simulink model "TransformadaZ"  (R2017b)
settings: Solver=ode4  StartTime=0.0  StopTime=10.0  FixedStep=0.0001  RelTol=1e-3
settings Model: Creator=Benjamin Nicolas  LastModifiedBy=Benjamin Nicolas

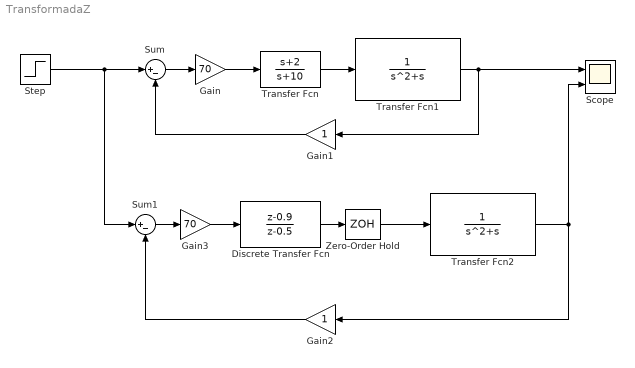
== system TransformadaZ ==
  Discrete Transfer Fcn : DiscreteTransferFcn  Numerator=[1 -0.9]  Denominator=[1 -0.5]  SampleTime=0.05
  Gain : Gain  Gain=70
  Gain1 : Gain
  Gain2 : Gain
  Gain3 : Gain  Gain=70
  Scope : Scope  NumInputPorts=2
  Step : Step  Time=0  SampleTime=10
  Sum : Sum  Inputs=|+-
  Sum1 : Sum  Inputs=|+-
  Transfer Fcn : TransferFcn  Numerator=[1 2]  Denominator=[1 10]
  Transfer Fcn1 : TransferFcn  Denominator=[1 1 0]
  Transfer Fcn2 : TransferFcn  Denominator=[1 1 0]
  Zero-Order Hold : ZeroOrderHold  SampleTime=-1
  wires:
  Gain/1 -> Transfer Fcn/1
  Transfer Fcn/1 -> Transfer Fcn1/1
  Transfer Fcn1/1 -> Scope/1, Gain1/1
  Step/1 -> Sum/1, Sum1/1
  Sum/1 -> Gain/1
  Gain1/1 -> Sum/2
  Gain2/1 -> Sum1/2
  Sum1/1 -> Gain3/1
  Gain3/1 -> Discrete Transfer Fcn/1
  Discrete Transfer Fcn/1 -> Zero-Order Hold/1
  Transfer Fcn2/1 -> Gain2/1, Scope/2
  Zero-Order Hold/1 -> Transfer Fcn2/1
